simulink model "TEST_IPM_2_0"  (R2019b)
settings: configuration reference "Configuration" (kept outside this file)
PreLoadFcn:
  | RTWConfigurationCB('preloadfcn', bdroot);
values from neighbouring files (symbols this model uses):
  MParamFbase = 200.0    [TEST_IPM_LIB.sldd]
  MParamIbase = 360.0    [TEST_IPM_LIB.sldd]
  MParamLd = 0.002    [TEST_IPM_LIB.sldd]
  MParamLq = 0.002    [TEST_IPM_LIB.sldd]
  MParamRs = 1.15    [TEST_IPM_LIB.sldd]
  PWM_TPBRD_HALF = 5000.0    [TEST_IPM_LIB.sldd]
  Ts_10kHz = 0.0001    [TEST_IPM_LIB.sldd]
  Ts_1kHz = 0.001    [TEST_IPM_LIB.sldd]
undefined symbols (not defined in the file or in its folder): Down, GPTRIP1SEL, GPTRIP2SEL, TZ1, TZ2, Up
libraries: c280xlib x66, c2837xDlib x18, c2802xlib x10, powerlib_meascontrol x9, dsparch4 x4, c2000lib x1, c2806xlib x1, idelinklib_common x1
(part 4 of 6)

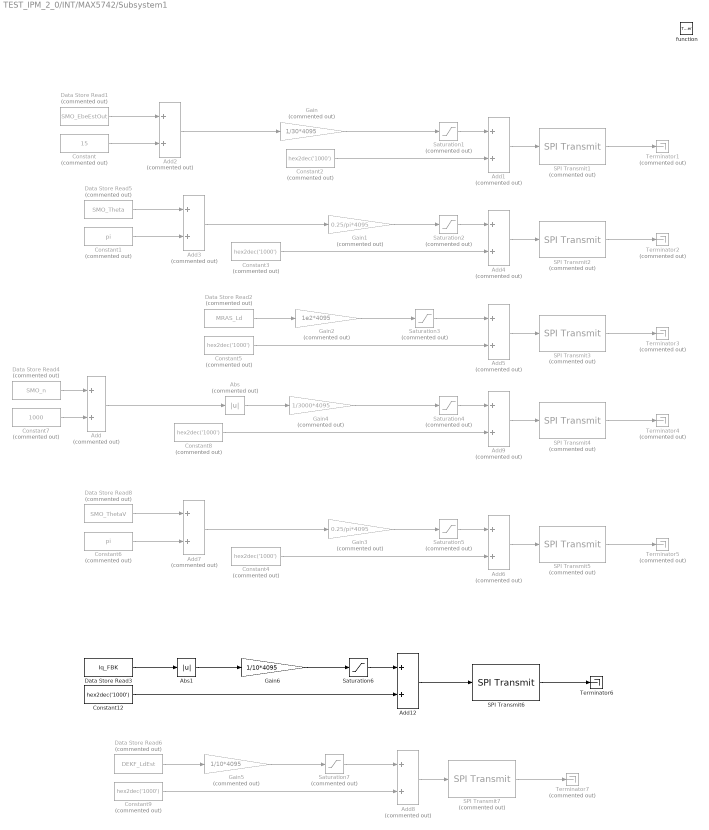
== system TEST_IPM_2_0/INT/MAX5742/Subsystem1 ==
  function : TriggerPort  TriggerType=function-call  VariantControl=Variant
  Abs : Abs  Commented=on
  Abs1 : Abs
  Add{,1..9} (10 alike) : Sum  Commented=on
  Add12 : Sum
  Constant : Constant  Commented=on  Value=15  OutDataTypeStr=single  SampleTime=-1
  Constant1 : Constant  Commented=on  Value=pi  OutDataTypeStr=single  SampleTime=-1
  Constant12 : Constant  Value=hex2dec('1000')  OutDataTypeStr=uint16  SampleTime=-1
  Constant{2..5,8..9} (6 alike) : Constant  Commented=on  Value=hex2dec('1000')  OutDataTypeStr=uint16  SampleTime=-1
  Constant6 : Constant  Commented=on  Value=pi  OutDataTypeStr=single  SampleTime=-1
  Constant7 : Constant  Commented=on  Value=1000  OutDataTypeStr=single  SampleTime=-1
  Data Store Read1 : DataStoreRead  Commented=on  DataStoreName=SMO_EbeEstOut
  Data Store Read2 : DataStoreRead  Commented=on  DataStoreName=MRAS_Ld
  Data Store Read3 : DataStoreRead  DataStoreName=Iq_FBK
  Data Store Read4 : DataStoreRead  Commented=on  DataStoreName=SMO_n
  Data Store Read5 : DataStoreRead  Commented=on  DataStoreName=SMO_Theta
  Data Store Read6 : DataStoreRead  Commented=on  DataStoreName=DEKF_LdEst
  Data Store Read8 : DataStoreRead  Commented=on  DataStoreName=SMO_ThetaV
  Gain : Gain  Commented=on  Gain=1/30*4095
  Gain1 : Gain  Commented=on  Gain=0.25/pi*4095
  Gain2 : Gain  Commented=on  Gain=1e2*4095
  Gain3 : Gain  Commented=on  Gain=0.25/pi*4095
  Gain4 : Gain  Commented=on  Gain=1/3000*4095
  Gain5 : Gain  Commented=on  Gain=1/10*4095
  Gain6 : Gain  Gain=1/10*4095
  SPI Transmit{1..5,7} (6 alike) : c280xlib/SPI Transmit  Commented=on  SPISelect=SPI_B  ClockPolarity=Rising_edge  ClockPhase=No_delay  SPIModule=uint32(0)  Mode=Master  BusSpeed=uint32(1000000)  FirstBitToTransfer=Most significant bit (MSB)  ClockMode=0  BlockFunction=Write  EnableRegisterAddress=on  RegisterAddress=0  OutputDataType=int8  OutputDataLength=1  BlockingMode=off  DataBits=16  UseCustomSSPin=Provided by the SPI peripheral  ActiveLowSSPin=Active low  Pin=0
      settings: SourceProductName=Embedded Coder Support Package for Texas Instruments C2000 Processors  SourceProductBaseCode=TIC2000
  SPI Transmit6 : c280xlib/SPI Transmit  SPISelect=SPI_B  ClockPolarity=Rising_edge  ClockPhase=No_delay  SPIModule=uint32(0)  Mode=Master  BusSpeed=uint32(1000000)  FirstBitToTransfer=Most significant bit (MSB)  ClockMode=0  BlockFunction=Write  EnableRegisterAddress=on  RegisterAddress=0  OutputDataType=int8  OutputDataLength=1  BlockingMode=off  DataBits=16  UseCustomSSPin=Provided by the SPI peripheral  ActiveLowSSPin=Active low  Pin=0
      settings: SourceProductName=Embedded Coder Support Package for Texas Instruments C2000 Processors  SourceProductBaseCode=TIC2000
  Saturation{1..5,7} (6 alike) : Saturate  Commented=on  UpperLimit=4095  LowerLimit=0  OutDataTypeStr=uint16
  Saturation6 : Saturate  UpperLimit=4095  LowerLimit=0  OutDataTypeStr=uint16
  Terminator{1..5,7} (6 alike) : Terminator  Commented=on
  Terminator6 : Terminator
  wires:
  Saturation1/1 -> Add1/1
  Add1/1 -> SPI Transmit1/1
  SPI Transmit1/1 -> Terminator1/1
  Constant2/1 -> Add1/2
  Gain/1 -> Saturation1/1
  Data Store Read1/1 -> Add2/1
  Constant/1 -> Add2/2
  Add2/1 -> Gain/1
  Constant3/1 -> Add4/2
  Add4/1 -> SPI Transmit2/1
  Saturation2/1 -> Add4/1
  Gain1/1 -> Saturation2/1
  Data Store Read5/1 -> Add3/1
  Constant1/1 -> Add3/2
  Add3/1 -> Gain1/1
  SPI Transmit2/1 -> Terminator2/1
  Saturation3/1 -> Add5/1
  SPI Transmit3/1 -> Terminator3/1
  Add5/1 -> SPI Transmit3/1
  Gain2/1 -> Saturation3/1
  Constant5/1 -> Add5/2
  Data Store Read2/1 -> Gain2/1
  SPI Transmit4/1 -> Terminator4/1
  Add9/1 -> SPI Transmit4/1
  Saturation4/1 -> Add9/1
  Constant8/1 -> Add9/2
  Gain4/1 -> Saturation4/1
  Constant7/1 -> Add/2
  Data Store Read4/1 -> Add/1
  Abs/1 -> Gain4/1
  Add/1 -> Abs/1
  Saturation5/1 -> Add6/1
  Constant6/1 -> Add7/2
  Constant4/1 -> Add6/2
  Add7/1 -> Gain3/1
  Gain3/1 -> Saturation5/1
  SPI Transmit5/1 -> Terminator5/1
  Add6/1 -> SPI Transmit5/1
  Data Store Read8/1 -> Add7/1
  Gain6/1 -> Saturation6/1
  Constant12/1 -> Add12/2
  Saturation6/1 -> Add12/1
  Abs1/1 -> Gain6/1
  Data Store Read3/1 -> Abs1/1
  Add12/1 -> SPI Transmit6/1
  SPI Transmit6/1 -> Terminator6/1
  SPI Transmit7/1 -> Terminator7/1
  Data Store Read6/1 -> Gain5/1
  Gain5/1 -> Saturation7/1
  Constant9/1 -> Add8/2
  Saturation7/1 -> Add8/1
  Add8/1 -> SPI Transmit7/1

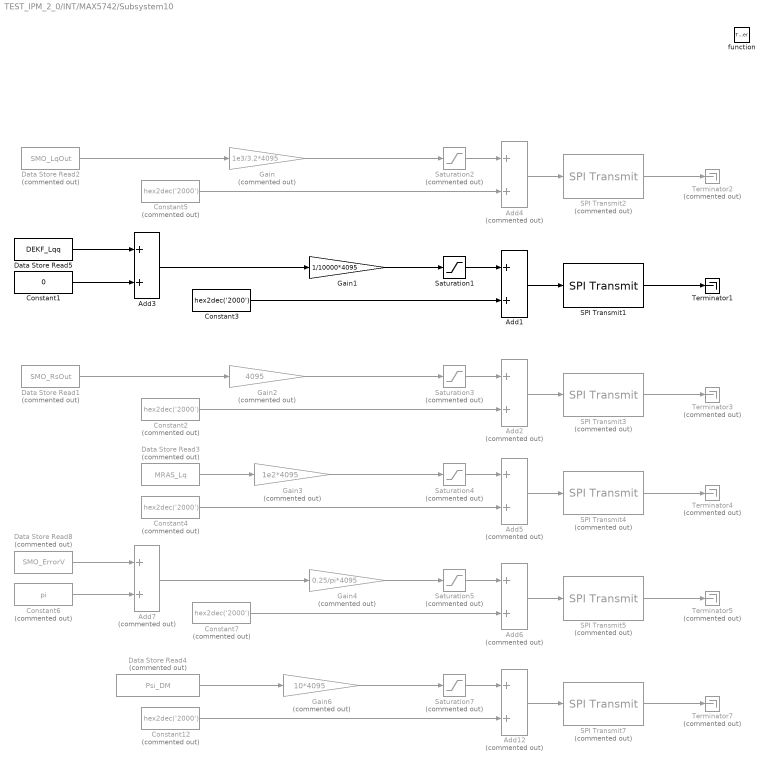
== system TEST_IPM_2_0/INT/MAX5742/Subsystem10 ==
  function : TriggerPort  TriggerType=function-call  VariantControl=Variant
  Add1 : Sum
  Add{2,4..7,12} (6 alike) : Sum  Commented=on
  Add3 : Sum
  Constant1 : Constant  Value=0  OutDataTypeStr=single  SampleTime=-1
  Constant{2,4..5,7,12} (5 alike) : Constant  Commented=on  Value=hex2dec('2000')  OutDataTypeStr=uint16  SampleTime=-1
  Constant3 : Constant  Value=hex2dec('2000')  OutDataTypeStr=uint16  SampleTime=-1
  Constant6 : Constant  Commented=on  Value=pi  OutDataTypeStr=single  SampleTime=-1
  Data Store Read1 : DataStoreRead  Commented=on  DataStoreName=SMO_RsOut
  Data Store Read2 : DataStoreRead  Commented=on  DataStoreName=SMO_LqOut
  Data Store Read3 : DataStoreRead  Commented=on  DataStoreName=MRAS_Lq
  Data Store Read4 : DataStoreRead  Commented=on  DataStoreName=Psi_DM
  Data Store Read5 : DataStoreRead  DataStoreName=DEKF_Lqq
  Data Store Read8 : DataStoreRead  Commented=on  DataStoreName=SMO_ErrorV
  Gain : Gain  Commented=on  Gain=1e3/3.2*4095
  Gain1 : Gain  Gain=1/10000*4095
  Gain2 : Gain  Commented=on  Gain=4095
  Gain3 : Gain  Commented=on  Gain=1e2*4095
  Gain4 : Gain  Commented=on  Gain=0.25/pi*4095
  Gain6 : Gain  Commented=on  Gain=10*4095
  SPI Transmit1 : c280xlib/SPI Transmit  SPISelect=SPI_B  ClockPolarity=Rising_edge  ClockPhase=No_delay  SPIModule=uint32(0)  Mode=Master  BusSpeed=uint32(1000000)  FirstBitToTransfer=Most significant bit (MSB)  ClockMode=0  BlockFunction=Write  EnableRegisterAddress=on  RegisterAddress=0  OutputDataType=int8  OutputDataLength=1  BlockingMode=off  DataBits=16  UseCustomSSPin=Provided by the SPI peripheral  ActiveLowSSPin=Active low  Pin=0
      settings: SourceProductName=Embedded Coder Support Package for Texas Instruments C2000 Processors  SourceProductBaseCode=TIC2000
  SPI Transmit{2..5,7} (5 alike) : c280xlib/SPI Transmit  Commented=on  SPISelect=SPI_B  ClockPolarity=Rising_edge  ClockPhase=No_delay  SPIModule=uint32(0)  Mode=Master  BusSpeed=uint32(1000000)  FirstBitToTransfer=Most significant bit (MSB)  ClockMode=0  BlockFunction=Write  EnableRegisterAddress=on  RegisterAddress=0  OutputDataType=int8  OutputDataLength=1  BlockingMode=off  DataBits=16  UseCustomSSPin=Provided by the SPI peripheral  ActiveLowSSPin=Active low  Pin=0
      settings: SourceProductName=Embedded Coder Support Package for Texas Instruments C2000 Processors  SourceProductBaseCode=TIC2000
  Saturation1 : Saturate  UpperLimit=4095  LowerLimit=0  OutDataTypeStr=uint16
  Saturation{2..5,7} (5 alike) : Saturate  Commented=on  UpperLimit=4095  LowerLimit=0  OutDataTypeStr=uint16
  Terminator1 : Terminator
  Terminator{2..5,7} (5 alike) : Terminator  Commented=on
  wires:
  Saturation4/1 -> Add5/1
  Constant4/1 -> Add5/2
  SPI Transmit4/1 -> Terminator4/1
  Gain3/1 -> Saturation4/1
  Add5/1 -> SPI Transmit4/1
  Data Store Read3/1 -> Gain3/1
  SPI Transmit3/1 -> Terminator3/1
  Add2/1 -> SPI Transmit3/1
  Gain2/1 -> Saturation3/1
  Saturation3/1 -> Add2/1
  Data Store Read1/1 -> Gain2/1
  Constant2/1 -> Add2/2
  Data Store Read2/1 -> Gain/1
  Gain/1 -> Saturation2/1
  SPI Transmit2/1 -> Terminator2/1
  Add4/1 -> SPI Transmit2/1
  Saturation2/1 -> Add4/1
  Constant5/1 -> Add4/2
  Constant1/1 -> Add3/2
  Data Store Read5/1 -> Add3/1
  Saturation1/1 -> Add1/1
  Add3/1 -> Gain1/1
  Gain1/1 -> Saturation1/1
  Add1/1 -> SPI Transmit1/1
  SPI Transmit1/1 -> Terminator1/1
  Constant3/1 -> Add1/2
  SPI Transmit5/1 -> Terminator5/1
  Data Store Read8/1 -> Add7/1
  Constant6/1 -> Add7/2
  Add7/1 -> Gain4/1
  Constant7/1 -> Add6/2
  Saturation5/1 -> Add6/1
  Gain4/1 -> Saturation5/1
  Add6/1 -> SPI Transmit5/1
  Add12/1 -> SPI Transmit7/1
  Saturation7/1 -> Add12/1
  Constant12/1 -> Add12/2
  Data Store Read4/1 -> Gain6/1
  SPI Transmit7/1 -> Terminator7/1
  Gain6/1 -> Saturation7/1

== system TEST_IPM_2_0/INT/MAX5742/Subsystem11 ==
  function : TriggerPort  TriggerType=function-call  VariantControl=Variant
  Add{3..5,12} (4 alike) : Sum  Commented=on
  Add6 : Sum
  Add7 : Sum
  Constant1 : Constant  Value=pi  OutDataTypeStr=single  SampleTime=-1
  Constant12 : Constant  Commented=on  Value=hex2dec('3000')  OutDataTypeStr=uint16  SampleTime=-1
  Constant3 : Constant  Commented=on  Value=2048  OutDataTypeStr=single  SampleTime=-1
  Constant4 : Constant  Commented=on  Value=hex2dec('3000')  OutDataTypeStr=uint16  SampleTime=-1
  Constant6 : Constant  Commented=on  Value=hex2dec('3000')  OutDataTypeStr=uint16  SampleTime=-1
  Constant7 : Constant  Value=hex2dec('3000')  OutDataTypeStr=uint16  SampleTime=-1
  Data Store Read : DataStoreRead  Commented=on  DataStoreName=DEKF_PsiEst
  Data Store Read2 : DataStoreRead  Commented=on  DataStoreName=SMO_LqOut
  Data Store Read3 : DataStoreRead  Commented=on  DataStoreName=MRAS_Ldq
  Data Store Read8 : DataStoreRead  DataStoreName=SMO_ErrorV
  Gain : Gain  Commented=on  Gain=1e3/3.2*4095
  Gain3 : Gain  Commented=on  Gain=1e2*4095
  Gain4 : Gain  Gain=0.25/pi*4095
  Gain6 : Gain  Commented=on  Gain=1/100*4095
  SPI Transmit3 : c280xlib/SPI Transmit  Commented=on  SPISelect=SPI_B  ClockPolarity=Rising_edge  ClockPhase=No_delay  SPIModule=uint32(0)  Mode=Master  BusSpeed=uint32(1000000)  FirstBitToTransfer=Most significant bit (MSB)  ClockMode=0  BlockFunction=Write  EnableRegisterAddress=on  RegisterAddress=0  OutputDataType=int8  OutputDataLength=1  BlockingMode=off  DataBits=16  UseCustomSSPin=Provided by the SPI peripheral  ActiveLowSSPin=Active low  Pin=0
      settings: SourceProductName=Embedded Coder Support Package for Texas Instruments C2000 Processors  SourceProductBaseCode=TIC2000
  SPI Transmit4 : c280xlib/SPI Transmit  Commented=on  SPISelect=SPI_B  ClockPolarity=Rising_edge  ClockPhase=No_delay  SPIModule=uint32(0)  Mode=Master  BusSpeed=uint32(1000000)  FirstBitToTransfer=Most significant bit (MSB)  ClockMode=0  BlockFunction=Write  EnableRegisterAddress=on  RegisterAddress=0  OutputDataType=int8  OutputDataLength=1  BlockingMode=off  DataBits=16  UseCustomSSPin=Provided by the SPI peripheral  ActiveLowSSPin=Active low  Pin=0
      settings: SourceProductName=Embedded Coder Support Package for Texas Instruments C2000 Processors  SourceProductBaseCode=TIC2000
  SPI Transmit5 : c280xlib/SPI Transmit  SPISelect=SPI_B  ClockPolarity=Rising_edge  ClockPhase=No_delay  SPIModule=uint32(0)  Mode=Master  BusSpeed=uint32(1000000)  FirstBitToTransfer=Most significant bit (MSB)  ClockMode=0  BlockFunction=Write  EnableRegisterAddress=on  RegisterAddress=0  OutputDataType=int8  OutputDataLength=1  BlockingMode=off  DataBits=16  UseCustomSSPin=Provided by the SPI peripheral  ActiveLowSSPin=Active low  Pin=0
      settings: SourceProductName=Embedded Coder Support Package for Texas Instruments C2000 Processors  SourceProductBaseCode=TIC2000
  SPI Transmit7 : c280xlib/SPI Transmit  Commented=on  SPISelect=SPI_B  ClockPolarity=Rising_edge  ClockPhase=No_delay  SPIModule=uint32(0)  Mode=Master  BusSpeed=uint32(1000000)  FirstBitToTransfer=Most significant bit (MSB)  ClockMode=0  BlockFunction=Write  EnableRegisterAddress=on  RegisterAddress=0  OutputDataType=int8  OutputDataLength=1  BlockingMode=off  DataBits=16  UseCustomSSPin=Provided by the SPI peripheral  ActiveLowSSPin=Active low  Pin=0
      settings: SourceProductName=Embedded Coder Support Package for Texas Instruments C2000 Processors  SourceProductBaseCode=TIC2000
  Saturation3 : Saturate  Commented=on  UpperLimit=4095  LowerLimit=0  OutDataTypeStr=uint16
  Saturation4 : Saturate  Commented=on  UpperLimit=4095  LowerLimit=0  OutDataTypeStr=uint16
  Saturation5 : Saturate  UpperLimit=4095  LowerLimit=0  OutDataTypeStr=uint16
  Saturation7 : Saturate  Commented=on  UpperLimit=4095  LowerLimit=0  OutDataTypeStr=uint16
  Terminator3 : Terminator  Commented=on
  Terminator4 : Terminator  Commented=on
  Terminator5 : Terminator
  Terminator7 : Terminator  Commented=on
  wires:
  Gain3/1 -> Add4/1
  Add4/1 -> Saturation4/1
  Constant3/1 -> Add4/2
  SPI Transmit4/1 -> Terminator4/1
  Data Store Read3/1 -> Gain3/1
  Add5/1 -> SPI Transmit4/1
  Saturation4/1 -> Add5/1
  Constant4/1 -> Add5/2
  Gain/1 -> Saturation3/1
  Data Store Read2/1 -> Gain/1
  Add3/1 -> SPI Transmit3/1
  Saturation3/1 -> Add3/1
  Constant6/1 -> Add3/2
  SPI Transmit3/1 -> Terminator3/1
  Add6/1 -> SPI Transmit5/1
  Add7/1 -> Gain4/1
  Data Store Read8/1 -> Add7/1
  Saturation5/1 -> Add6/1
  SPI Transmit5/1 -> Terminator5/1
  Gain4/1 -> Saturation5/1
  Constant1/1 -> Add7/2
  Constant7/1 -> Add6/2
  Constant12/1 -> Add12/2
  SPI Transmit7/1 -> Terminator7/1
  Gain6/1 -> Saturation7/1
  Data Store Read/1 -> Gain6/1
  Saturation7/1 -> Add12/1
  Add12/1 -> SPI Transmit7/1

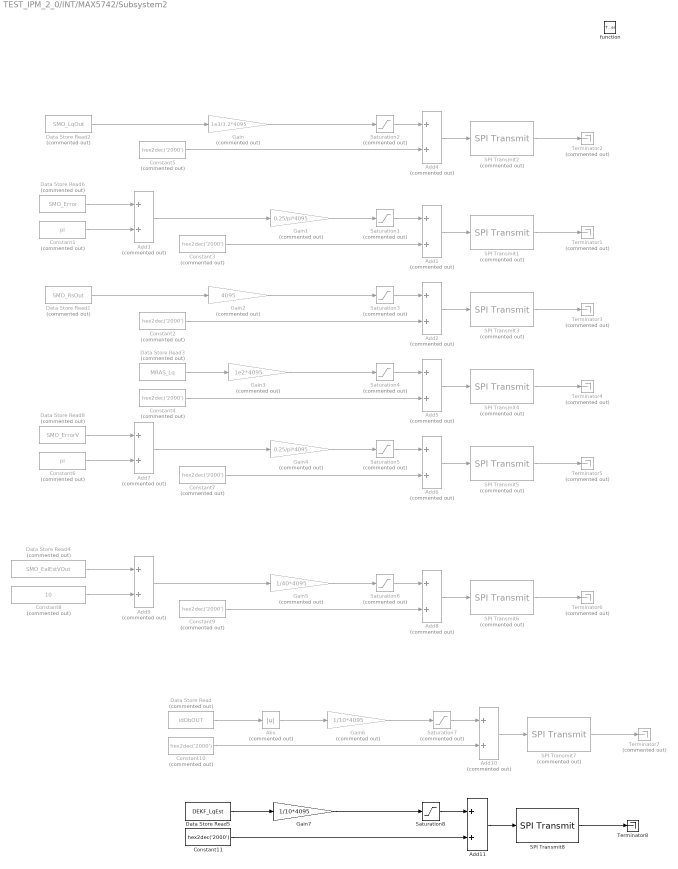
== system TEST_IPM_2_0/INT/MAX5742/Subsystem2 ==
  function : TriggerPort  TriggerType=function-call  VariantControl=Variant
  Abs : Abs  Commented=on
  Add{1..10} (10 alike) : Sum  Commented=on
  Add11 : Sum
  Constant1 : Constant  Commented=on  Value=pi  OutDataTypeStr=single  SampleTime=-1
  Constant{2..5,7,9..10} (7 alike) : Constant  Commented=on  Value=hex2dec('2000')  OutDataTypeStr=uint16  SampleTime=-1
  Constant11 : Constant  Value=hex2dec('2000')  OutDataTypeStr=uint16  SampleTime=-1
  Constant6 : Constant  Commented=on  Value=pi  OutDataTypeStr=single  SampleTime=-1
  Constant8 : Constant  Commented=on  Value=10  OutDataTypeStr=single  SampleTime=-1
  Data Store Read : DataStoreRead  Commented=on  DataStoreName=idObOUT
  Data Store Read1 : DataStoreRead  Commented=on  DataStoreName=SMO_RsOut
  Data Store Read2 : DataStoreRead  Commented=on  DataStoreName=SMO_LqOut
  Data Store Read3 : DataStoreRead  Commented=on  DataStoreName=MRAS_Lq
  Data Store Read4 : DataStoreRead  Commented=on  DataStoreName=SMO_EalEstVOut
  Data Store Read5 : DataStoreRead  DataStoreName=DEKF_LqEst
  Data Store Read6 : DataStoreRead  Commented=on  DataStoreName=SMO_Error
  Data Store Read8 : DataStoreRead  Commented=on  DataStoreName=SMO_ErrorV
  Gain : Gain  Commented=on  Gain=1e3/3.2*4095
  Gain1 : Gain  Commented=on  Gain=0.25/pi*4095
  Gain2 : Gain  Commented=on  Gain=4095
  Gain3 : Gain  Commented=on  Gain=1e2*4095
  Gain4 : Gain  Commented=on  Gain=0.25/pi*4095
  Gain5 : Gain  Commented=on  Gain=1/40*4095
  Gain6 : Gain  Commented=on  Gain=1/10*4095
  Gain7 : Gain  Gain=1/10*4095
  SPI Transmit{1..7} (7 alike) : c280xlib/SPI Transmit  Commented=on  SPISelect=SPI_B  ClockPolarity=Rising_edge  ClockPhase=No_delay  SPIModule=uint32(0)  Mode=Master  BusSpeed=uint32(1000000)  FirstBitToTransfer=Most significant bit (MSB)  ClockMode=0  BlockFunction=Write  EnableRegisterAddress=on  RegisterAddress=0  OutputDataType=int8  OutputDataLength=1  BlockingMode=off  DataBits=16  UseCustomSSPin=Provided by the SPI peripheral  ActiveLowSSPin=Active low  Pin=0
      settings: SourceProductName=Embedded Coder Support Package for Texas Instruments C2000 Processors  SourceProductBaseCode=TIC2000
  SPI Transmit8 : c280xlib/SPI Transmit  SPISelect=SPI_B  ClockPolarity=Rising_edge  ClockPhase=No_delay  SPIModule=uint32(0)  Mode=Master  BusSpeed=uint32(1000000)  FirstBitToTransfer=Most significant bit (MSB)  ClockMode=0  BlockFunction=Write  EnableRegisterAddress=on  RegisterAddress=0  OutputDataType=int8  OutputDataLength=1  BlockingMode=off  DataBits=16  UseCustomSSPin=Provided by the SPI peripheral  ActiveLowSSPin=Active low  Pin=0
      settings: SourceProductName=Embedded Coder Support Package for Texas Instruments C2000 Processors  SourceProductBaseCode=TIC2000
  Saturation{1..7} (7 alike) : Saturate  Commented=on  UpperLimit=4095  LowerLimit=0  OutDataTypeStr=uint16
  Saturation8 : Saturate  UpperLimit=4095  LowerLimit=0  OutDataTypeStr=uint16
  Terminator{1..7} (7 alike) : Terminator  Commented=on
  Terminator8 : Terminator
  wires:
  Constant5/1 -> Add4/2
  Saturation2/1 -> Add4/1
  Add4/1 -> SPI Transmit2/1
  SPI Transmit2/1 -> Terminator2/1
  Gain/1 -> Saturation2/1
  Data Store Read2/1 -> Gain/1
  Gain1/1 -> Saturation1/1
  Constant3/1 -> Add1/2
  Constant1/1 -> Add3/2
  Saturation1/1 -> Add1/1
  Add3/1 -> Gain1/1
  Data Store Read6/1 -> Add3/1
  Add1/1 -> SPI Transmit1/1
  SPI Transmit1/1 -> Terminator1/1
  Constant2/1 -> Add2/2
  Data Store Read1/1 -> Gain2/1
  Saturation3/1 -> Add2/1
  Gain2/1 -> Saturation3/1
  Add2/1 -> SPI Transmit3/1
  SPI Transmit3/1 -> Terminator3/1
  Data Store Read3/1 -> Gain3/1
  Add5/1 -> SPI Transmit4/1
  Gain3/1 -> Saturation4/1
  SPI Transmit4/1 -> Terminator4/1
  Constant4/1 -> Add5/2
  Saturation4/1 -> Add5/1
  Saturation5/1 -> Add6/1
  Data Store Read8/1 -> Add7/1
  Gain4/1 -> Saturation5/1
  Constant6/1 -> Add7/2
  Constant7/1 -> Add6/2
  Add7/1 -> Gain4/1
  SPI Transmit5/1 -> Terminator5/1
  Add6/1 -> SPI Transmit5/1
  Saturation6/1 -> Add8/1
  Constant9/1 -> Add8/2
  Gain5/1 -> Saturation6/1
  Data Store Read4/1 -> Add9/1
  SPI Transmit6/1 -> Terminator6/1
  Add9/1 -> Gain5/1
  Constant8/1 -> Add9/2
  Add8/1 -> SPI Transmit6/1
  Saturation7/1 -> Add10/1
  Gain6/1 -> Saturation7/1
  Abs/1 -> Gain6/1
  SPI Transmit7/1 -> Terminator7/1
  Add10/1 -> SPI Transmit7/1
  Constant10/1 -> Add10/2
  Data Store Read/1 -> Abs/1
  Saturation8/1 -> Add11/1
  Constant11/1 -> Add11/2
  Data Store Read5/1 -> Gain7/1
  Gain7/1 -> Saturation8/1
  SPI Transmit8/1 -> Terminator8/1
  Add11/1 -> SPI Transmit8/1

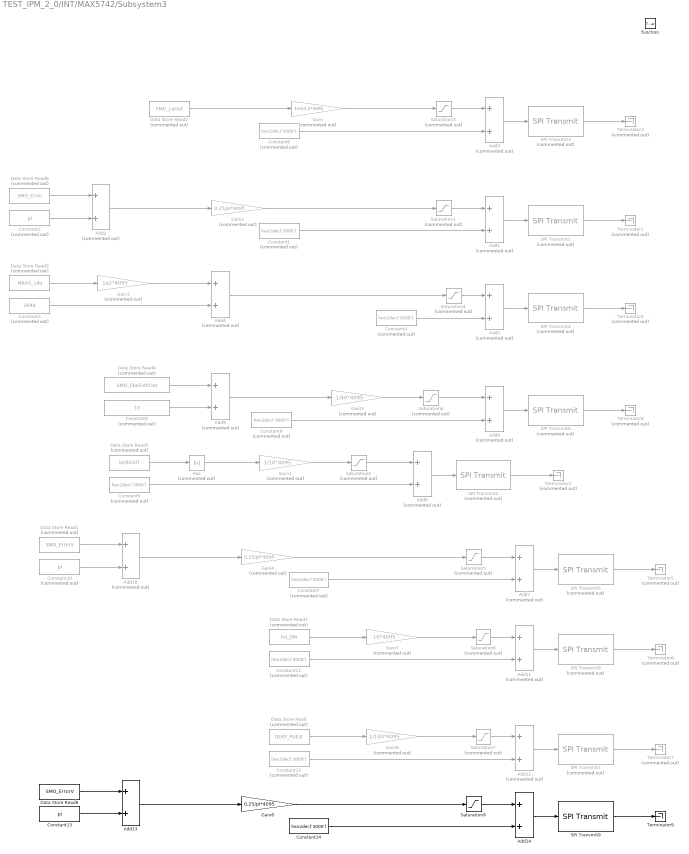
== system TEST_IPM_2_0/INT/MAX5742/Subsystem3 ==
  function : TriggerPort  TriggerType=function-call  VariantControl=Variant
  Abs : Abs  Commented=on
  Add{1..12} (12 alike) : Sum  Commented=on
  Add13 : Sum
  Add14 : Sum
  Constant{1,4..7,9,11..12} (8 alike) : Constant  Commented=on  Value=hex2dec('3000')  OutDataTypeStr=uint16  SampleTime=-1
  Constant10 : Constant  Commented=on  Value=pi  OutDataTypeStr=single  SampleTime=-1
  Constant13 : Constant  Value=pi  OutDataTypeStr=single  SampleTime=-1
  Constant14 : Constant  Value=hex2dec('3000')  OutDataTypeStr=uint16  SampleTime=-1
  Constant2 : Constant  Commented=on  Value=pi  OutDataTypeStr=single  SampleTime=-1
  Constant3 : Constant  Commented=on  Value=2048  OutDataTypeStr=single  SampleTime=-1
  Constant8 : Constant  Commented=on  Value=10  OutDataTypeStr=single  SampleTime=-1
  Data Store Read : DataStoreRead  Commented=on  DataStoreName=DEKF_PsiEst
  Data Store Read1 : DataStoreRead  Commented=on  DataStoreName=SMO_ErrorV
  Data Store Read2 : DataStoreRead  Commented=on  DataStoreName=SMO_LqOut
  Data Store Read3 : DataStoreRead  Commented=on  DataStoreName=MRAS_Ldq
  Data Store Read4 : DataStoreRead  Commented=on  DataStoreName=SMO_EbeEstVOut
  Data Store Read5 : DataStoreRead  Commented=on  DataStoreName=iqObOUT
  Data Store Read6 : DataStoreRead  Commented=on  DataStoreName=SMO_Error
  Data Store Read7 : DataStoreRead  Commented=on  DataStoreName=Psi_DM
  Data Store Read8 : DataStoreRead  DataStoreName=SMO_ErrorV
  Gain : Gain  Commented=on  Gain=1e3/3.2*4095
  Gain1 : Gain  Commented=on  Gain=1/10*4095
  Gain2 : Gain  Commented=on  Gain=0.25/pi*4095
  Gain3 : Gain  Commented=on  Gain=1e2*4095
  Gain4 : Gain  Commented=on  Gain=0.25/pi*4095
  Gain5 : Gain  Commented=on  Gain=1/40*4095
  Gain6 : Gain  Commented=on  Gain=1/100*4095
  Gain7 : Gain  Commented=on  Gain=10*4095
  Gain8 : Gain  Gain=0.25/pi*4095
  SPI Transmit{1..8} (8 alike) : c280xlib/SPI Transmit  Commented=on  SPISelect=SPI_B  ClockPolarity=Rising_edge  ClockPhase=No_delay  SPIModule=uint32(0)  Mode=Master  BusSpeed=uint32(1000000)  FirstBitToTransfer=Most significant bit (MSB)  ClockMode=0  BlockFunction=Write  EnableRegisterAddress=on  RegisterAddress=0  OutputDataType=int8  OutputDataLength=1  BlockingMode=off  DataBits=16  UseCustomSSPin=Provided by the SPI peripheral  ActiveLowSSPin=Active low  Pin=0
      settings: SourceProductName=Embedded Coder Support Package for Texas Instruments C2000 Processors  SourceProductBaseCode=TIC2000
  SPI Transmit9 : c280xlib/SPI Transmit  SPISelect=SPI_B  ClockPolarity=Rising_edge  ClockPhase=No_delay  SPIModule=uint32(0)  Mode=Master  BusSpeed=uint32(1000000)  FirstBitToTransfer=Most significant bit (MSB)  ClockMode=0  BlockFunction=Write  EnableRegisterAddress=on  RegisterAddress=0  OutputDataType=int8  OutputDataLength=1  BlockingMode=off  DataBits=16  UseCustomSSPin=Provided by the SPI peripheral  ActiveLowSSPin=Active low  Pin=0
      settings: SourceProductName=Embedded Coder Support Package for Texas Instruments C2000 Processors  SourceProductBaseCode=TIC2000
  Saturation{1..8} (8 alike) : Saturate  Commented=on  UpperLimit=4095  LowerLimit=0  OutDataTypeStr=uint16
  Saturation9 : Saturate  UpperLimit=4095  LowerLimit=0  OutDataTypeStr=uint16
  Terminator{1..8} (8 alike) : Terminator  Commented=on
  Terminator9 : Terminator
  wires:
  SPI Transmit3/1 -> Terminator3/1
  Constant6/1 -> Add3/2
  Saturation3/1 -> Add3/1
  Add3/1 -> SPI Transmit3/1
  Data Store Read2/1 -> Gain/1
  Gain/1 -> Saturation3/1
  Constant1/1 -> Add1/2
  Add1/1 -> SPI Transmit1/1
  Saturation1/1 -> Add1/1
  Gain2/1 -> Saturation1/1
  SPI Transmit1/1 -> Terminator1/1
  Add2/1 -> Gain2/1
  Data Store Read6/1 -> Add2/1
  Constant2/1 -> Add2/2
  Constant4/1 -> Add5/2
  Saturation4/1 -> Add5/1
  Add5/1 -> SPI Transmit4/1
  Data Store Read3/1 -> Gain3/1
  SPI Transmit4/1 -> Terminator4/1
  Constant3/1 -> Add4/2
  Add4/1 -> Saturation4/1
  Gain3/1 -> Add4/1
  Add8/1 -> SPI Transmit6/1
  Constant8/1 -> Add9/2
  SPI Transmit6/1 -> Terminator6/1
  Gain5/1 -> Saturation6/1
  Constant9/1 -> Add8/2
  Add9/1 -> Gain5/1
  Saturation6/1 -> Add8/1
  Data Store Read4/1 -> Add9/1
  Gain1/1 -> Saturation2/1
  Data Store Read5/1 -> Abs/1
  Constant5/1 -> Add6/2
  SPI Transmit2/1 -> Terminator2/1
  Add6/1 -> SPI Transmit2/1
  Saturation2/1 -> Add6/1
  Abs/1 -> Gain1/1
  Saturation5/1 -> Add7/1
  SPI Transmit5/1 -> Terminator5/1
  Constant7/1 -> Add7/2
  Constant10/1 -> Add10/2
  Data Store Read1/1 -> Add10/1
  Add7/1 -> SPI Transmit5/1
  Gain4/1 -> Saturation5/1
  Add10/1 -> Gain4/1
  SPI Transmit8/1 -> Terminator8/1
  Add11/1 -> SPI Transmit8/1
  Data Store Read7/1 -> Gain7/1
  Saturation8/1 -> Add11/1
  Constant11/1 -> Add11/2
  Gain7/1 -> Saturation8/1
  Constant12/1 -> Add12/2
  Saturation7/1 -> Add12/1
  Add12/1 -> SPI Transmit7/1
  Gain6/1 -> Saturation7/1
  Data Store Read/1 -> Gain6/1
  SPI Transmit7/1 -> Terminator7/1
  Constant13/1 -> Add13/2
  Constant14/1 -> Add14/2
  Data Store Read8/1 -> Add13/1
  Add14/1 -> SPI Transmit9/1
  Saturation9/1 -> Add14/1
  Add13/1 -> Gain8/1
  SPI Transmit9/1 -> Terminator9/1
  Gain8/1 -> Saturation9/1

== system TEST_IPM_2_0/INT/MAX5742/Subsystem4 ==
  function : TriggerPort  TriggerType=function-call  VariantControl=Variant
  Add2 : Sum
  Constant1 : Constant  Value=hex2dec('0000')  OutDataTypeStr=uint16  SampleTime=-1
  Constant2 : Constant  Priority=102  Value=1024  OutDataTypeStr=Inherit: Inherit via back propagation  SampleTime=-1
  SPI Transmit : c280xlib/SPI Transmit  SPISelect=SPI_B  ClockPolarity=Rising_edge  ClockPhase=No_delay  SPIModule=uint32(0)  Mode=Master  BusSpeed=uint32(1000000)  FirstBitToTransfer=Most significant bit (MSB)  ClockMode=0  BlockFunction=Write  EnableRegisterAddress=on  RegisterAddress=0  OutputDataType=int8  OutputDataLength=1  BlockingMode=off  DataBits=16  UseCustomSSPin=Provided by the SPI peripheral  ActiveLowSSPin=Active low  Pin=0
      settings: SourceProductName=Embedded Coder Support Package for Texas Instruments C2000 Processors  SourceProductBaseCode=TIC2000
  Saturation : Saturate  UpperLimit=4095  LowerLimit=0  OutDataTypeStr=uint16
  Terminator : Terminator
  wires:
  Constant1/1 -> Add2/2
  SPI Transmit/1 -> Terminator/1
  Saturation/1 -> Add2/1
  Constant2/1 -> Saturation/1
  Add2/1 -> SPI Transmit/1

== system TEST_IPM_2_0/INT/MAX5742/Subsystem5 ==
  function : TriggerPort  TriggerType=function-call  VariantControl=Variant
  Add1 : Sum
  Constant1 : Constant  Priority=107  Value=2048  OutDataTypeStr=Inherit: Inherit via back propagation  SampleTime=-1
  Constant2 : Constant  Value=hex2dec('1000')  OutDataTypeStr=uint16  SampleTime=-1
  SPI Transmit1 : c280xlib/SPI Transmit  SPISelect=SPI_B  ClockPolarity=Rising_edge  ClockPhase=No_delay  SPIModule=uint32(0)  Mode=Master  BusSpeed=uint32(1000000)  FirstBitToTransfer=Most significant bit (MSB)  ClockMode=0  BlockFunction=Write  EnableRegisterAddress=on  RegisterAddress=0  OutputDataType=int8  OutputDataLength=1  BlockingMode=off  DataBits=16  UseCustomSSPin=Provided by the SPI peripheral  ActiveLowSSPin=Active low  Pin=0
      settings: SourceProductName=Embedded Coder Support Package for Texas Instruments C2000 Processors  SourceProductBaseCode=TIC2000
  Saturation1 : Saturate  UpperLimit=4095  LowerLimit=0  OutDataTypeStr=uint16
  Terminator1 : Terminator
  wires:
  Saturation1/1 -> Add1/1
  Add1/1 -> SPI Transmit1/1
  SPI Transmit1/1 -> Terminator1/1
  Constant2/1 -> Add1/2
  Constant1/1 -> Saturation1/1

== system TEST_IPM_2_0/INT/MAX5742/Subsystem6 ==
  function : TriggerPort  TriggerType=function-call  VariantControl=Variant
  Add4 : Sum
  Constant1 : Constant  Priority=112  Value=3072  OutDataTypeStr=Inherit: Inherit via back propagation  SampleTime=-1
  Constant5 : Constant  Value=hex2dec('2000')  OutDataTypeStr=uint16  SampleTime=-1
  SPI Transmit2 : c280xlib/SPI Transmit  SPISelect=SPI_B  ClockPolarity=Rising_edge  ClockPhase=No_delay  SPIModule=uint32(0)  Mode=Master  BusSpeed=uint32(1000000)  FirstBitToTransfer=Most significant bit (MSB)  ClockMode=0  BlockFunction=Write  EnableRegisterAddress=on  RegisterAddress=0  OutputDataType=int8  OutputDataLength=1  BlockingMode=off  DataBits=16  UseCustomSSPin=Provided by the SPI peripheral  ActiveLowSSPin=Active low  Pin=0
      settings: SourceProductName=Embedded Coder Support Package for Texas Instruments C2000 Processors  SourceProductBaseCode=TIC2000
  Saturation2 : Saturate  UpperLimit=4095  LowerLimit=0  OutDataTypeStr=uint16
  Terminator2 : Terminator
  wires:
  Constant5/1 -> Add4/2
  Saturation2/1 -> Add4/1
  Add4/1 -> SPI Transmit2/1
  SPI Transmit2/1 -> Terminator2/1
  Constant1/1 -> Saturation2/1

== system TEST_IPM_2_0/INT/MAX5742/Subsystem7 ==
  function : TriggerPort  TriggerType=function-call  VariantControl=Variant
  Add3 : Sum
  Constant6 : Constant  Value=hex2dec('3000')  OutDataTypeStr=uint16  SampleTime=-1
  Data Store Read : DataStoreRead  DataStoreName=UDCPROTECT
  SPI Transmit3 : c280xlib/SPI Transmit  SPISelect=SPI_B  ClockPolarity=Rising_edge  ClockPhase=No_delay  SPIModule=uint32(0)  Mode=Master  BusSpeed=uint32(1000000)  FirstBitToTransfer=Most significant bit (MSB)  ClockMode=0  BlockFunction=Write  EnableRegisterAddress=on  RegisterAddress=0  OutputDataType=int8  OutputDataLength=1  BlockingMode=off  DataBits=16  UseCustomSSPin=Provided by the SPI peripheral  ActiveLowSSPin=Active low  Pin=0
      settings: SourceProductName=Embedded Coder Support Package for Texas Instruments C2000 Processors  SourceProductBaseCode=TIC2000
  Saturation3 : Saturate  UpperLimit=4095  LowerLimit=0  OutDataTypeStr=uint16
  Terminator3 : Terminator
  wires:
  SPI Transmit3/1 -> Terminator3/1
  Constant6/1 -> Add3/2
  Data Store Read/1 -> Saturation3/1
  Saturation3/1 -> Add3/1
  Add3/1 -> SPI Transmit3/1

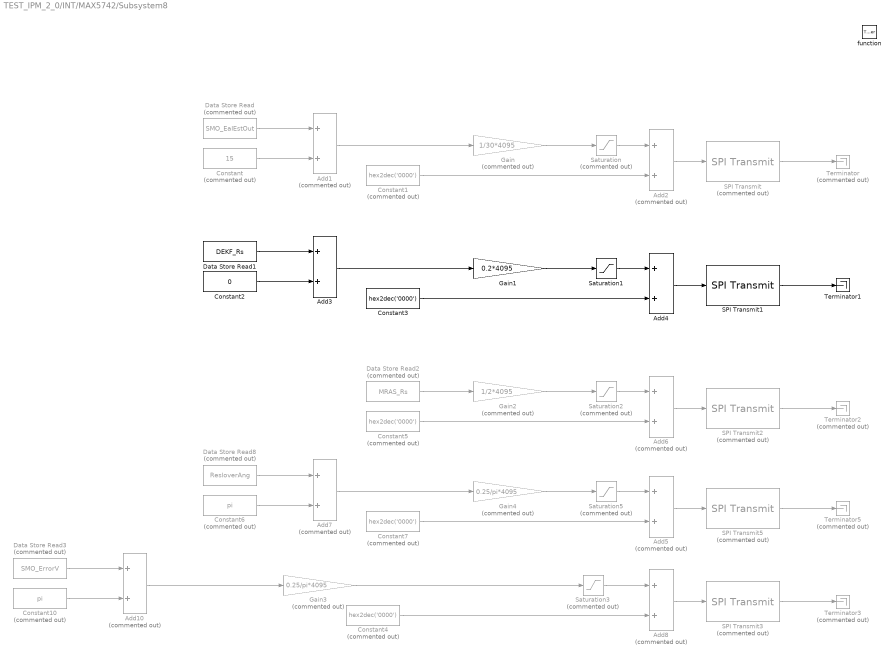
== system TEST_IPM_2_0/INT/MAX5742/Subsystem8 ==
  function : TriggerPort  TriggerType=function-call  VariantControl=Variant
  Add{1..2,5..8,10} (7 alike) : Sum  Commented=on
  Add3 : Sum
  Add4 : Sum
  Constant : Constant  Commented=on  Value=15  OutDataTypeStr=single  SampleTime=-1
  Constant{1,4..5,7} (4 alike) : Constant  Commented=on  Value=hex2dec('0000')  OutDataTypeStr=uint16  SampleTime=-1
  Constant10 : Constant  Commented=on  Value=pi  OutDataTypeStr=single  SampleTime=-1
  Constant2 : Constant  Value=0  OutDataTypeStr=single  SampleTime=-1
  Constant3 : Constant  Value=hex2dec('0000')  OutDataTypeStr=uint16  SampleTime=-1
  Constant6 : Constant  Commented=on  Value=pi  OutDataTypeStr=single  SampleTime=-1
  Data Store Read : DataStoreRead  Commented=on  DataStoreName=SMO_EalEstOut
  Data Store Read1 : DataStoreRead  DataStoreName=DEKF_Rs
  Data Store Read2 : DataStoreRead  Commented=on  DataStoreName=MRAS_Rs
  Data Store Read3 : DataStoreRead  Commented=on  DataStoreName=SMO_ErrorV
  Data Store Read8 : DataStoreRead  Commented=on  DataStoreName=ResloverAng
  Gain : Gain  Commented=on  Gain=1/30*4095
  Gain1 : Gain  Gain=0.2*4095
  Gain2 : Gain  Commented=on  Gain=1/2*4095
  Gain3 : Gain  Commented=on  Gain=0.25/pi*4095
  Gain4 : Gain  Commented=on  Gain=0.25/pi*4095
  SPI Transmit{,2..3,5} (4 alike) : c280xlib/SPI Transmit  Commented=on  SPISelect=SPI_B  ClockPolarity=Rising_edge  ClockPhase=No_delay  SPIModule=uint32(0)  Mode=Master  BusSpeed=uint32(1000000)  FirstBitToTransfer=Most significant bit (MSB)  ClockMode=0  BlockFunction=Write  EnableRegisterAddress=on  RegisterAddress=0  OutputDataType=int8  OutputDataLength=1  BlockingMode=off  DataBits=16  UseCustomSSPin=Provided by the SPI peripheral  ActiveLowSSPin=Active low  Pin=0
      settings: SourceProductName=Embedded Coder Support Package for Texas Instruments C2000 Processors  SourceProductBaseCode=TIC2000
  SPI Transmit1 : c280xlib/SPI Transmit  SPISelect=SPI_B  ClockPolarity=Rising_edge  ClockPhase=No_delay  SPIModule=uint32(0)  Mode=Master  BusSpeed=uint32(1000000)  FirstBitToTransfer=Most significant bit (MSB)  ClockMode=0  BlockFunction=Write  EnableRegisterAddress=on  RegisterAddress=0  OutputDataType=int8  OutputDataLength=1  BlockingMode=off  DataBits=16  UseCustomSSPin=Provided by the SPI peripheral  ActiveLowSSPin=Active low  Pin=0
      settings: SourceProductName=Embedded Coder Support Package for Texas Instruments C2000 Processors  SourceProductBaseCode=TIC2000
  Saturation{,2..3,5} (4 alike) : Saturate  Commented=on  UpperLimit=4095  LowerLimit=0  OutDataTypeStr=uint16
  Saturation1 : Saturate  UpperLimit=4095  LowerLimit=0  OutDataTypeStr=uint16
  Terminator{,2..3,5} (4 alike) : Terminator  Commented=on
  Terminator1 : Terminator
  wires:
  Data Store Read2/1 -> Gain2/1
  Add6/1 -> SPI Transmit2/1
  Gain2/1 -> Saturation2/1
  SPI Transmit2/1 -> Terminator2/1
  Saturation2/1 -> Add6/1
  Constant5/1 -> Add6/2
  Data Store Read1/1 -> Add3/1
  Constant2/1 -> Add3/2
  Add3/1 -> Gain1/1
  Add4/1 -> SPI Transmit1/1
  Constant3/1 -> Add4/2
  SPI Transmit1/1 -> Terminator1/1
  Saturation1/1 -> Add4/1
  Gain1/1 -> Saturation1/1
  Constant/1 -> Add1/2
  Data Store Read/1 -> Add1/1
  Add1/1 -> Gain/1
  Gain/1 -> Saturation/1
  Add2/1 -> SPI Transmit/1
  Saturation/1 -> Add2/1
  SPI Transmit/1 -> Terminator/1
  Constant1/1 -> Add2/2
  Saturation5/1 -> Add5/1
  Constant7/1 -> Add5/2
  Gain4/1 -> Saturation5/1
  Data Store Read8/1 -> Add7/1
  SPI Transmit5/1 -> Terminator5/1
  Add7/1 -> Gain4/1
  Constant6/1 -> Add7/2
  Add5/1 -> SPI Transmit5/1
  Add8/1 -> SPI Transmit3/1
  Data Store Read3/1 -> Add10/1
  SPI Transmit3/1 -> Terminator3/1
  Saturation3/1 -> Add8/1
  Add10/1 -> Gain3/1
  Constant10/1 -> Add10/2
  Constant4/1 -> Add8/2
  Gain3/1 -> Saturation3/1

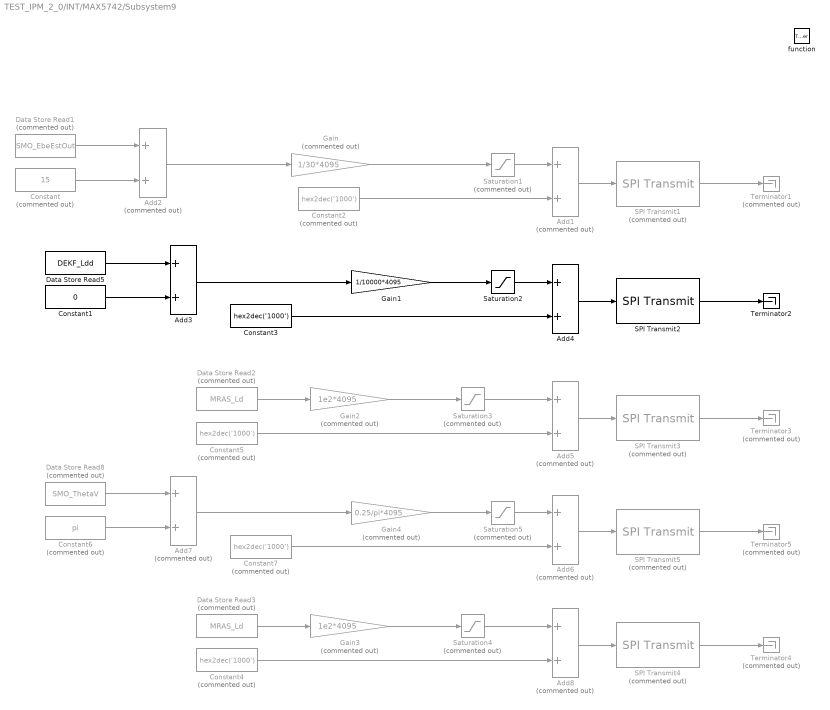
== system TEST_IPM_2_0/INT/MAX5742/Subsystem9 ==
  function : TriggerPort  TriggerType=function-call  VariantControl=Variant
  Add{1..2,5..8} (6 alike) : Sum  Commented=on
  Add3 : Sum
  Add4 : Sum
  Constant : Constant  Commented=on  Value=15  OutDataTypeStr=single  SampleTime=-1
  Constant1 : Constant  Value=0  OutDataTypeStr=single  SampleTime=-1
  Constant{2,4..5,7} (4 alike) : Constant  Commented=on  Value=hex2dec('1000')  OutDataTypeStr=uint16  SampleTime=-1
  Constant3 : Constant  Value=hex2dec('1000')  OutDataTypeStr=uint16  SampleTime=-1
  Constant6 : Constant  Commented=on  Value=pi  OutDataTypeStr=single  SampleTime=-1
  Data Store Read1 : DataStoreRead  Commented=on  DataStoreName=SMO_EbeEstOut
  Data Store Read2 : DataStoreRead  Commented=on  DataStoreName=MRAS_Ld
  Data Store Read3 : DataStoreRead  Commented=on  DataStoreName=MRAS_Ld
  Data Store Read5 : DataStoreRead  DataStoreName=DEKF_Ldd
  Data Store Read8 : DataStoreRead  Commented=on  DataStoreName=SMO_ThetaV
  Gain : Gain  Commented=on  Gain=1/30*4095
  Gain1 : Gain  Gain=1/10000*4095
  Gain2 : Gain  Commented=on  Gain=1e2*4095
  Gain3 : Gain  Commented=on  Gain=1e2*4095
  Gain4 : Gain  Commented=on  Gain=0.25/pi*4095
  SPI Transmit{1,3..5} (4 alike) : c280xlib/SPI Transmit  Commented=on  SPISelect=SPI_B  ClockPolarity=Rising_edge  ClockPhase=No_delay  SPIModule=uint32(0)  Mode=Master  BusSpeed=uint32(1000000)  FirstBitToTransfer=Most significant bit (MSB)  ClockMode=0  BlockFunction=Write  EnableRegisterAddress=on  RegisterAddress=0  OutputDataType=int8  OutputDataLength=1  BlockingMode=off  DataBits=16  UseCustomSSPin=Provided by the SPI peripheral  ActiveLowSSPin=Active low  Pin=0
      settings: SourceProductName=Embedded Coder Support Package for Texas Instruments C2000 Processors  SourceProductBaseCode=TIC2000
  SPI Transmit2 : c280xlib/SPI Transmit  SPISelect=SPI_B  ClockPolarity=Rising_edge  ClockPhase=No_delay  SPIModule=uint32(0)  Mode=Master  BusSpeed=uint32(1000000)  FirstBitToTransfer=Most significant bit (MSB)  ClockMode=0  BlockFunction=Write  EnableRegisterAddress=on  RegisterAddress=0  OutputDataType=int8  OutputDataLength=1  BlockingMode=off  DataBits=16  UseCustomSSPin=Provided by the SPI peripheral  ActiveLowSSPin=Active low  Pin=0
      settings: SourceProductName=Embedded Coder Support Package for Texas Instruments C2000 Processors  SourceProductBaseCode=TIC2000
  Saturation{1,3..5} (4 alike) : Saturate  Commented=on  UpperLimit=4095  LowerLimit=0  OutDataTypeStr=uint16
  Saturation2 : Saturate  UpperLimit=4095  LowerLimit=0  OutDataTypeStr=uint16
  Terminator{1,3..5} (4 alike) : Terminator  Commented=on
  Terminator2 : Terminator
  wires:
  Data Store Read2/1 -> Gain2/1
  Constant5/1 -> Add5/2
  Gain2/1 -> Saturation3/1
  Add5/1 -> SPI Transmit3/1
  SPI Transmit3/1 -> Terminator3/1
  Saturation3/1 -> Add5/1
  SPI Transmit2/1 -> Terminator2/1
  Add3/1 -> Gain1/1
  Constant1/1 -> Add3/2
  Data Store Read5/1 -> Add3/1
  Gain1/1 -> Saturation2/1
  Saturation2/1 -> Add4/1
  Add4/1 -> SPI Transmit2/1
  Constant3/1 -> Add4/2
  Add2/1 -> Gain/1
  Constant/1 -> Add2/2
  Data Store Read1/1 -> Add2/1
  Gain/1 -> Saturation1/1
  Constant2/1 -> Add1/2
  SPI Transmit1/1 -> Terminator1/1
  Add1/1 -> SPI Transmit1/1
  Saturation1/1 -> Add1/1
  SPI Transmit5/1 -> Terminator5/1
  Data Store Read8/1 -> Add7/1
  Constant6/1 -> Add7/2
  Add7/1 -> Gain4/1
  Constant7/1 -> Add6/2
  Saturation5/1 -> Add6/1
  Gain4/1 -> Saturation5/1
  Add6/1 -> SPI Transmit5/1
  Gain3/1 -> Saturation4/1
  SPI Transmit4/1 -> Terminator4/1
  Constant4/1 -> Add8/2
  Saturation4/1 -> Add8/1
  Add8/1 -> SPI Transmit4/1
  Data Store Read3/1 -> Gain3/1

== system TEST_IPM_2_0/INT/Motor Control/Adjusting Mode ==
  Action Port : ActionPort  ActionPortLabel=case [ 0 ]:

== system TEST_IPM_2_0/INT/Motor Control/Clark Transformation ==
  U : Inport
  V : Inport  Port=2
  W : Inport  Port=3
  Add : Sum  Inputs=+--
  Add1 : Sum  Inputs=+-
  Gain : Gain  Gain=0.5
  Gain1 : Gain  Gain=0.5
  Gain2 : Gain  Gain=2/3
  Gain3 : Gain  Gain=2/3*0.86602540
  Alpha : Outport
  Beta : Outport  Port=2
  wires:
  V/1 -> Add1/1, Gain/1
  Gain/1 -> Add/2
  W/1 -> Add1/2, Gain1/1
  Gain1/1 -> Add/3
  U/1 -> Add/1
  Add/1 -> Gain2/1
  Gain2/1 -> Alpha/1
  Add1/1 -> Gain3/1
  Gain3/1 -> Beta/1

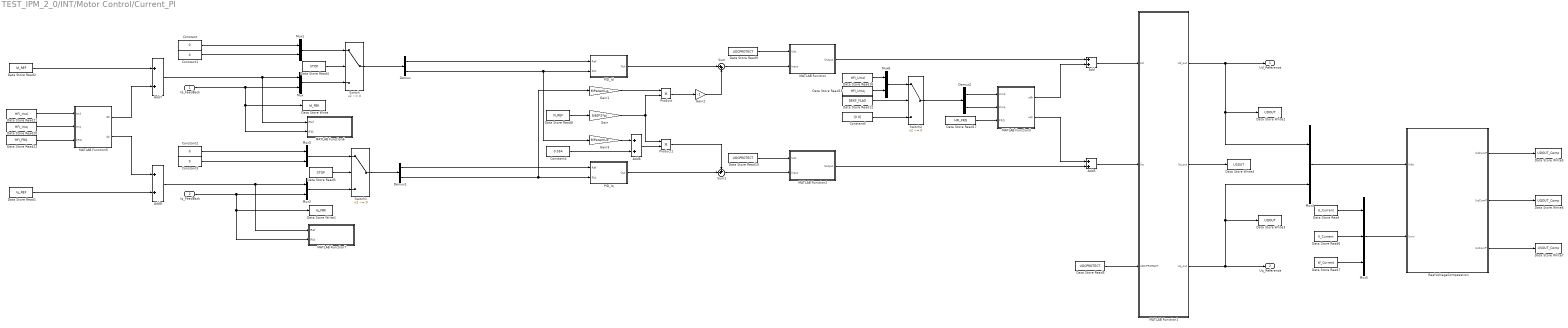
== system TEST_IPM_2_0/INT/Motor Control/Current_PI ==
  Id_FeedBack : Inport
  Iq_FeedBack : Inport  Port=2
  Add{,5..8} (5 alike) : Sum
  Constant{,1..3} (4 alike) : Constant  Value=0  OutDataTypeStr=single  SampleTime=-1
  Constant4 : Constant  Value=0.054  OutDataTypeStr=single  SampleTime=-1
  Constant5 : Constant  Value=[0 0]  OutDataTypeStr=single  SampleTime=-1
  Data Store Read : DataStoreRead  DataStoreName=U_Current
  Data Store Read1 : DataStoreRead  DataStoreName=Iq_REF
  Data Store Read10 : DataStoreRead  DataStoreName=UDCPROTECT
  Data Store Read12 : DataStoreRead  DataStoreName=DEKF_FLAG
  Data Store Read15 : DataStoreRead  DataStoreName=HFI_Umq
  Data Store Read16 : DataStoreRead  DataStoreName=HFI_Umd
  Data Store Read17 : DataStoreRead  DataStoreName=HFI_FRQ
  Data Store Read2 : DataStoreRead  DataStoreName=Id_REF
  Data Store Read20 : DataStoreRead  DataStoreName=HFI_Imq
  Data Store Read21 : DataStoreRead  DataStoreName=HFI_Imd
  Data Store Read22 : DataStoreRead  DataStoreName=HFI_FRQ
  Data Store Read3 : DataStoreRead  DataStoreName=STOP
  Data Store Read4 : DataStoreRead  DataStoreName=STOP
  Data Store Read5 : DataStoreRead  DataStoreName=UDCPROTECT
  Data Store Read6 : DataStoreRead  DataStoreName=V_Current
  Data Store Read7 : DataStoreRead  DataStoreName=W_Current
  Data Store Read8 : DataStoreRead  DataStoreName=N_REF
  Data Store Read9 : DataStoreRead  DataStoreName=UDCPROTECT
  Data Store Write : DataStoreWrite  DataStoreName=Id_FBK
  Data Store Write1 : DataStoreWrite  DataStoreName=Iq_FBK
  Data Store Write2 : DataStoreWrite  DataStoreName=UDOUT
  Data Store Write3 : DataStoreWrite  DataStoreName=UQOUT
  Data Store Write4 : DataStoreWrite  DataStoreName=USOUT
  Data Store Write5 : DataStoreWrite  DataStoreName=UDOUT_Comp
  Data Store Write6 : DataStoreWrite  DataStoreName=UQOUT_Comp
  Data Store Write7 : DataStoreWrite  DataStoreName=USOUT_Comp
  Demux : Demux  Outputs=2
  Demux1 : Demux  Outputs=2
  Demux2 : Demux  Outputs=2
  Gain : Gain  Gain=5/60*2*pi
  Gain1 : Gain  Gain=MParamLq
  Gain2 : Gain  Gain=-1
  Gain3 : Gain  Gain=MParamLd
  MATLAB Function : MATLAB Function  TreatAsAtomicUnit=on
  MATLAB Function1 : MATLAB Function  TreatAsAtomicUnit=on
  MATLAB Function2 : MATLAB Function  TreatAsAtomicUnit=on
  MATLAB Function3 : MATLAB Function  TreatAsAtomicUnit=on
  MATLAB Function5 : MATLAB Function  TreatAsAtomicUnit=on
  MATLAB Function6 : MATLAB Function  TreatAsAtomicUnit=on
  MATLAB Function7 : MATLAB Function  TreatAsAtomicUnit=on
  Mux{,1..4,6} (6 alike) : Mux  Inputs=2
  Mux5 : Mux  Inputs=3
  "PID_Id " : Subsystem  TreatAsAtomicUnit=on
  PID_Iq : Subsystem  TreatAsAtomicUnit=on
  Product : Product
  Product1 : Product
  "RealVoltageCompesation " : Subsystem  TreatAsAtomicUnit=on
  Sum : Sum  Inputs=|++  AccumDataTypeStr=single
  Sum1 : Sum  Inputs=++|  AccumDataTypeStr=single
  Switch : Switch  Criteria=u2 ~= 0
  Switch1 : Switch  Criteria=u2 ~= 0
  Switch2 : Switch  Criteria=u2 ~= 0
  Ud_Reference : Outport
  Uq_Reference : Outport  Port=2
  wires:
  Mux/1 -> Switch/3
  Constant1/1 -> Mux1/2
  Mux1/1 -> Switch/1
  Data Store Read4/1 -> Switch/2
  Switch/1 -> Demux/1
  Constant/1 -> Mux1/1
  Demux1/1 -> PID_Iq/1(Ref)
  Switch1/1 -> Demux1/1
  Mux3/1 -> Switch1/1
  Constant2/1 -> Mux3/1
  Constant3/1 -> Mux3/2
  Mux2/1 -> Switch1/3
  Data Store Read3/1 -> Switch1/2
  Add8/1 -> MATLAB Function7/1(IRef), Mux2/1
  MATLAB Function1/1(Ud_out) -> Ud_Reference/1, Data Store Write2/1, Mux4/1
  MATLAB Function1/3(Uq_out) -> Uq_Reference/1, Mux4/2, Data Store Write3/1
  Iq_FeedBack/1 -> MATLAB Function7/2(IFbk), Data Store Write1/1, Mux2/2
  Id_FeedBack/1 -> Data Store Write/1, MATLAB Function6/2(IFbk), Mux/2
  MATLAB Function1/2(Us_out) -> Data Store Write4/1
  Data Store Read5/1 -> MATLAB Function1/3(UDCPROTECT)
  Mux4/1 -> "RealVoltageCompesation "/1(Udq)
  Mux5/1 -> "RealVoltageCompesation "/2(Iuvw)
  Data Store Read/1 -> Mux5/1
  Data Store Read6/1 -> Mux5/2
  Data Store Read7/1 -> Mux5/3
  "PID_Id "/1(Out) -> Sum/1
  PID_Iq/1(Out) -> Sum1/2
  Product/1 -> Gain2/1
  Data Store Read8/1 -> Gain/1
  Gain/1 -> Product1/1, Product/2
  Gain1/1 -> Product/1
  Gain2/1 -> Sum/2
  Data Store Read9/1 -> MATLAB Function/1(Udc)
  Sum/1 -> MATLAB Function/2(Input)
  Sum1/1 -> MATLAB Function2/2(Input)
  Data Store Read10/1 -> MATLAB Function2/1(Udc)
  Demux2/1 -> MATLAB Function3/1(Umd)
  Demux2/2 -> MATLAB Function3/2(Umq)
  Data Store Read17/1 -> MATLAB Function3/3(FRQ)
  MATLAB Function3/1(udh) -> Add/2
  MATLAB Function3/2(uqh) -> Add5/1
  Add/1 -> MATLAB Function1/1(Ud)
  Add5/1 -> MATLAB Function1/2(Uq)
  Product1/1 -> Sum1/1
  Add6/1 -> Product1/2
  Gain3/1 -> Add6/1
  Constant4/1 -> Add6/2
  Data Store Read22/1 -> MATLAB Function5/3(FRQ)
  Data Store Read20/1 -> MATLAB Function5/2(Imq)
  Data Store Read21/1 -> MATLAB Function5/1(Imd)
  Data Store Read2/1 -> Add7/1
  Add7/1 -> MATLAB Function6/1(IRef), Mux/1
  MATLAB Function5/1(idh) -> Add7/2
  Data Store Read1/1 -> Add8/2
  MATLAB Function5/2(iqh) -> Add8/1
  "RealVoltageCompesation "/2(UqComP) -> Data Store Write6/1
  "RealVoltageCompesation "/3(UsComP) -> Data Store Write7/1
  "RealVoltageCompesation "/1(UdComP) -> Data Store Write5/1
  Demux/1 -> "PID_Id "/1(Ref)
  MATLAB Function/1(Output) -> Add/1
  MATLAB Function2/1(Output) -> Add5/2
  Data Store Read12/1 -> Switch2/2
  Switch2/1 -> Demux2/1
  Mux6/1 -> Switch2/1
  Constant5/1 -> Switch2/3
  Data Store Read16/1 -> Mux6/1
  Data Store Read15/1 -> Mux6/2
  Demux/2 -> Gain3/1, "PID_Id "/2(Fbk)
  Demux1/2 -> Gain1/1, PID_Iq/2(Fbk)

== system TEST_IPM_2_0/INT/Motor Control/Error ==
  Action Port : ActionPort  ActionPortLabel=default:
  Constant : Constant  OutDataTypeStr=Inherit: Inherit via back propagation  SampleTime=-1
  Constant1 : Constant  Value=0  OutDataTypeStr=Inherit: Inherit via back propagation  SampleTime=-1
  Data Store Write1 : DataStoreWrite  DataStoreName=PROTECT
  Data Store Write2 : DataStoreWrite  DataStoreName=STOP
  wires:
  Constant/1 -> Data Store Write2/1
  Constant1/1 -> Data Store Write1/1

== system TEST_IPM_2_0/INT/Motor Control/IF ==
  Action Port : ActionPort  ActionPortLabel=case [ 2 ]:
  Data Store Read2 : DataStoreRead  DataStoreName=IF_F
  Data Store Read3 : DataStoreRead  DataStoreName=IF_F_Step
  Data Store Write : DataStoreWrite  DataStoreName=ControlAng
  Subsystem1 : Subsystem
  Subsystem2 : Subsystem
  wires:
  Data Store Read3/1 -> Subsystem1/2(Step)
  Data Store Read2/1 -> Subsystem1/1(TargetValue)
  Subsystem2/1(Ang) -> Data Store Write/1
  Subsystem1/1(RampOutput) -> Subsystem2/1(FRQ)

== system TEST_IPM_2_0/INT/Motor Control/Park Transformation ==
  Alpha : Inport
  Beta : Inport  Port=2
  theta : Inport  Port=3
  Add : Sum
  Add1 : Sum  Inputs=+-
  Product{,1..3} (4 alike) : Product
  Sin : Trigonometry  OutputSignalType=real
  Sin1 : Trigonometry  Operator=cos  OutputSignalType=real
  D : Outport
  Q : Outport  Port=2
  wires:
  Product/1 -> Add/1
  Sin/1 -> Product3/2, Product1/2
  Product1/1 -> Add/2
  Add1/1 -> Q/1
  Sin1/1 -> Product2/2, Product/2
  Product2/1 -> Add1/1
  Alpha/1 -> Product3/1, Product/1
  Beta/1 -> Product2/1, Product1/1
  Product3/1 -> Add1/2
  Add/1 -> D/1
  theta/1 -> Sin/1, Sin1/1

== system TEST_IPM_2_0/INT/Motor Control/SVPWM ==
  note: 由于矿车控制器ePWMxA是下管，B是上管，所以add变成了++
  Ud_Reference : Inport
  Uq_Reference : Inport  Port=2
  Angle : Inport  Port=3
  Constant1 : Constant  Value=PWM_TPBRD_HALF  OutDataTypeStr=single  SampleTime=-1
  Data Store Read : DataStoreRead  DataStoreName=UDCPROTECT
  Demux : Demux  Outputs=2
  Divide : Product  Inputs=*/
  Gain : Gain  Gain=1/sqrt(3)
  Gain1 : Gain  Gain=PWM_TPBRD_HALF  OutDataTypeStr=single  ParamDataTypeStr=Inherit: Same as input
  Inverse Park Transformation : Subsystem
  MATLAB Function : MATLAB Function  TreatAsAtomicUnit=on
  Mux : Mux  Inputs=2
  Mux1 : Mux  Inputs=3
  Saturation : Saturate  UpperLimit=370  LowerLimit=10
  Sum1 : Sum  Inputs=|-+  OutDataTypeStr=uint16
  COMPARE : Outport
  wires:
  Angle/1 -> Inverse Park Transformation/3(theta)
  Inverse Park Transformation/1(Alpha) -> MATLAB Function/1(alpha)
  Inverse Park Transformation/2(Beta) -> MATLAB Function/2(beta)
  Mux1/1 -> Gain1/1
  Sum1/1 -> COMPARE/1
  Gain1/1 -> Sum1/1
  Constant1/1 -> Sum1/2
  MATLAB Function/3(tc) -> Mux1/3
  MATLAB Function/2(tb) -> Mux1/2
  MATLAB Function/1(ta) -> Mux1/1
  Ud_Reference/1 -> Mux/1
  Uq_Reference/1 -> Mux/2
  Mux/1 -> Divide/1
  Saturation/1 -> Divide/2
  Data Store Read/1 -> Gain/1
  Gain/1 -> Saturation/1
  Demux/1 -> Inverse Park Transformation/1(D)
  Demux/2 -> Inverse Park Transformation/2(Q)
  Divide/1 -> Demux/1

== system TEST_IPM_2_0/INT/Motor Control/SpeedMode ==
  Action Port : ActionPort  ActionPortLabel=case [ 4 ]:
  Data Store Read : DataStoreRead  DataStoreName=SMO_AngControl_FLAG
  Data Store Read2 : DataStoreRead  DataStoreName=SMO_Theta
  Data Store Read3 : DataStoreRead  DataStoreName=N_REF
  Data Store Read4 : DataStoreRead  DataStoreName=ResloverAng
  Data Store Write1 : DataStoreWrite  DataStoreName=ControlAng
  Function-Call Subsystem : Subsystem  TreatAsAtomicUnit=on
  MATLAB Function : MATLAB Function  TreatAsAtomicUnit=on
  MATLAB Function1 : MATLAB Function  TreatAsAtomicUnit=on
  wires:
  MATLAB Function/1(Speed_PI()) -> Function-Call Subsystem/Trigger
  Data Store Read/1 -> MATLAB Function1/2(FLAG)
  MATLAB Function1/1(ThetaOut) -> Data Store Write1/1
  Data Store Read4/1 -> MATLAB Function1/3(ThetaReal)
  Data Store Read2/1 -> MATLAB Function1/1(ThetaEst)
  Data Store Read3/1 -> MATLAB Function1/4(nREF)

== system TEST_IPM_2_0/INT/Motor Control/Stop  ==
  Action Port : ActionPort  ActionPortLabel=case [ 5 ]:
  Constant3 : Constant  OutDataTypeStr=Inherit: Inherit via back propagation  SampleTime=-1
  Constant4 : Constant  Value=0  OutDataTypeStr=Inherit: Inherit via back propagation  SampleTime=-1
  Data Store Write3 : DataStoreWrite  DataStoreName=PROTECT
  Data Store Write4 : DataStoreWrite  DataStoreName=STOP
  wires:
  Constant3/1 -> Data Store Write4/1
  Constant4/1 -> Data Store Write3/1

== system TEST_IPM_2_0/INT/Motor Control/TorqueMode ==
  Action Port : ActionPort  ActionPortLabel=case [ 3 ]:
  Abs : Abs
  Data Store Read : DataStoreRead  DataStoreName=MTPA_Gamma
  Data Store Read1 : DataStoreRead  DataStoreName=Tem_Dem
  Data Store Read2 : DataStoreRead  DataStoreName=SMO_AngControl_FLAG
  Data Store Read3 : DataStoreRead  DataStoreName=Tem_Step
  Data Store Read4 : DataStoreRead  DataStoreName=N_FBK
  Data Store Read5 : DataStoreRead  DataStoreName=SMO_Theta
  Data Store Read6 : DataStoreRead  DataStoreName=N_REF
  Data Store Read7 : DataStoreRead  DataStoreName=ResloverAng
  Data Store Write1 : DataStoreWrite  DataStoreName=Iq_REF
  Data Store Write2 : DataStoreWrite  DataStoreName=Id_REF
  Data Store Write3 : DataStoreWrite  DataStoreName=ControlAng
  Function-Call Subsystem : Subsystem  TreatAsAtomicUnit=on
  Gain1 : Gain  Gain=-1  OutDataTypeStr=single
  MATLAB Function1 : MATLAB Function  TreatAsAtomicUnit=on
  MATLAB Function2 : MATLAB Function  TreatAsAtomicUnit=on
  MATLAB Function3 : MATLAB Function  TreatAsAtomicUnit=on
  Product : Product  OutDataTypeStr=single
  Product1 : Product  OutDataTypeStr=single
  Saturation : Saturate  UpperLimit=pi/2  LowerLimit=0
  cos : Trigonometry  Operator=cos  OutputSignalType=real
  sin : Trigonometry  OutputSignalType=real
  wires:
  Data Store Read1/1 -> MATLAB Function2/1(Target)
  Data Store Read3/1 -> MATLAB Function2/2(Step)
  Abs/1 -> Gain1/1
  Product/1 -> Data Store Write1/1
  Gain1/1 -> Product1/2
  Data Store Read4/1 -> MATLAB Function1/1(n)
  MATLAB Function1/1(PI_Clear()) -> Function-Call Subsystem/Trigger
  MATLAB Function2/1(Set_Point) -> Product/1, Abs/1
  Product1/1 -> Data Store Write2/1
  sin/1 -> Product1/1
  cos/1 -> Product/2
  Data Store Read/1 -> Saturation/1
  Saturation/1 -> sin/1, cos/1
  MATLAB Function3/1(ThetaOut) -> Data Store Write3/1
  Data Store Read2/1 -> MATLAB Function3/2(FLAG)
  Data Store Read6/1 -> MATLAB Function3/4(nREF)
  Data Store Read5/1 -> MATLAB Function3/1(ThetaEst)
  Data Store Read7/1 -> MATLAB Function3/3(ThetaReal)

== system TEST_IPM_2_0/INT/Motor Control/VF ==
  Action Port : ActionPort  ActionPortLabel=case [ 1 ]:
  Data Store Read : DataStoreRead  DataStoreName=VF_F
  Data Store Read2 : DataStoreRead  DataStoreName=VF_F_Step
  Data Store Write : DataStoreWrite  DataStoreName=ControlAng
  Subsystem1 : Subsystem
  Subsystem2 : Subsystem
  wires:
  Subsystem1/1(RampOutput) -> Subsystem2/1(FRQ)
  Subsystem2/1(Ang) -> Data Store Write/1
  Data Store Read/1 -> Subsystem1/1(TargetValue)
  Data Store Read2/1 -> Subsystem1/2(Step)

== system TEST_IPM_2_0/INT/Read Rotor Position/SpeedCal ==
  In1 : Inport
  function : TriggerPort  TriggerType=function-call  VariantControl=Variant
  "First Order Filter " : Subsystem
  MATLAB Function1 : MATLAB Function  TreatAsAtomicUnit=on
  Unit Delay : UnitDelay  SampleTime=-1  HasFrameUpgradeWarning=on
  Out1 : Outport
  wires:
  In1/1 -> Unit Delay/1, MATLAB Function1/1(theta)
  Unit Delay/1 -> MATLAB Function1/2(theta_old)
  MATLAB Function1/1(speed) -> "First Order Filter "/1(input)
  "First Order Filter "/1("output ") -> Out1/1
